simulink model "ex7p4"  (R2016b)
settings: Solver=VariableStepAuto  StartTime=0.0  StopTime=3  RelTol=1e-3
libraries: powerlib x9, simulink x1, powerlib_meascontrol x1
settings Model: Creator=user  LastModifiedBy=user

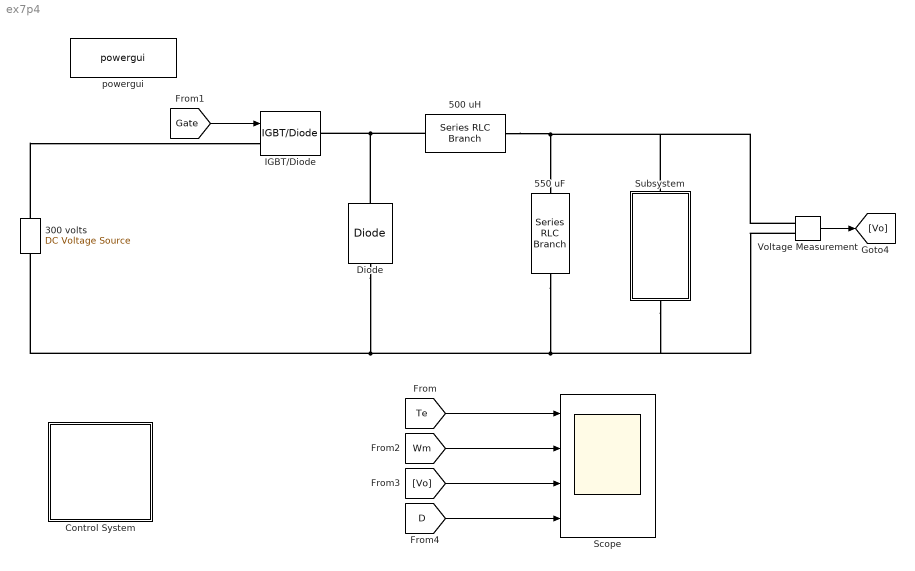
== system ex7p4 ==
  300 volts : powerlib/Electrical Sources/DC Voltage Source  Amplitude=300  Measurements=None
  500 uH : powerlib/Elements/Series RLC Branch  LConnTagsString=__new0  RConnTagsString=__new0  BranchType=L  Resistance=1  Inductance=500e-6  SetiL0=off  InitialCurrent=0  Capacitance=1e-6  Setx0=off  InitialVoltage=0  Measurements=None
  550 uF : powerlib/Elements/Series RLC Branch  LConnTagsString=__new0  RConnTagsString=__new0  BranchType=C  Resistance=1  Inductance=1e-3  SetiL0=off  InitialCurrent=0  Capacitance=550e-6  Setx0=on  InitialVoltage=150  Measurements=None
  "Control System " : Subsystem
  Diode : powerlib/Power Electronics/Diode  Ron=0.001  Lon=0  Vf=0.8  IC=0  UseSnubber=off  Rs=0  Cs=0  Measurements=off
  IGBT/Diode : powerlib/Power Electronics/IGBT//Diode  Ron=1e-3  Rs=1e5  Cs=inf  Measurements=off
  Scope : Scope  NumInputPorts=4
  Subsystem : Subsystem
  Voltage Measurement : powerlib/Measurements/Voltage Measurement  PhasorSimulation=off  OutputType=Complex  PSBequivalent=0
  powergui : powerlib/powergui  Priority=1  SimulationMode=Discrete  SolverType=Tustin/Backward Euler (TBE)  SampleTime=5e-6  frequency=60  SPID=off  DisableSnubberDevices=off  DisableRonSwitches=off  DisableVfSwitches=off  SwTol=0  DisplayEquations=off  Interpol=off  ExternalGateDelay=off  methode=off  Ts=10  FunctionMessages=off  echomessages=off  HookPort=off  EnableUseOfTLC=off  x0status=blocks  frequencyindice=0  Pbase=100e6  ErrMax=1e-4  Iterations=50  UnitsV=kV  UnitsW=MW  buscounter=0  RestoreLinks=warning  ResistiveCurrentMeasurement=off  Frange=[0:2:500]  Ylog=off  Xlog=on  ShowGrid=off  save=off  variable=ZData  structure=0  ZoomFFT=off  StartTime=0.0  cycles=1  DisplayStyle=1  fundamental=60  FreqAxis=off  MaxFrequency=1000  frequencyindicesteady=1  RmsSteady=1  display=off
  wires:
  Voltage Measurement/1 -> [Vo]
  [Te] -> Scope/1
  [Vo] -> Scope/3
  [D] -> Scope/4
  [Wm] -> Scope/2
  [Gate] -> IGBT/Diode/1
  connections:
  550 uF/RConn1 -- Subsystem/RConn1 -- Voltage Measurement/LConn2 -- Diode/LConn1 -- 300 volts/LConn1
  500 uH/LConn1 -- Subsystem/LConn1 -- Voltage Measurement/LConn1 -- 550 uF/LConn1
  300 volts/RConn1 -- IGBT/Diode/LConn1
  500 uH/RConn1 -- Diode/RConn1 -- IGBT/Diode/RConn1

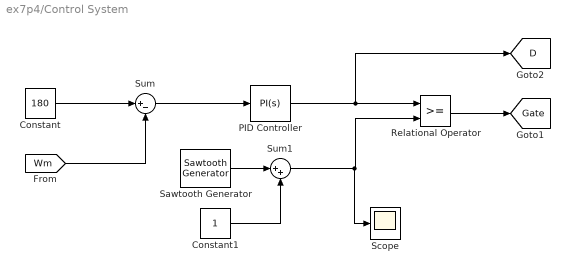
== system ex7p4/Control System  ==
  Constant : Constant  Value=180
  Constant1 : Constant
  PID Controller : simulink/Continuous/PID Controller  Controller=PI  TimeDomain=Continuous-time  SampleTime=-1  IntegratorMethod=Forward Euler  FilterMethod=Forward Euler  Form=Parallel  UseFilter=on  ControllerParametersSource=internal  P=0.1  I=2  D=0  N=100  InitialConditionSource=internal  InitialConditionForIntegrator=0  InitialConditionForFilter=0  ExternalReset=none  LimitOutput=off  UpperSaturationLimit=inf  LowerSaturationLimit=-inf  LinearizeAsGain=on  AntiWindupMode=none  Kb=1  TrackingMode=off  Kt=1  PParamMin=[]  PParamMax=[]  IParamMin=[]  IParamMax=[]  DParamMin=[]  DParamMax=[]  NParamMin=[]  NParamMax=[]  KbParamMin=[]  KbParamMax=[]  KtParamMin=[]  KtParamMax=[]  POutMin=[]  POutMax=[]  IOutMin=[]  IOutMax=[]  DOutMin=[]  DOutMax=[]  NOutMin=[]  NOutMax=[]  KbOutMin=[]  KbOutMax=[]  KtOutMin=[]  KtOutMax=[]  IntegratorOutMin=[]  IntegratorOutMax=[]  FilterOutMin=[]  FilterOutMax=[]  SumOutMin=[]  SumOutMax=[]  SumI1OutMin=[]  SumI1OutMax=[]  SumI2OutMin=[]  SumI2OutMax=[]  SumI3OutMin=[]  SumI3OutMax=[]  SumDOutMin=[]  SumDOutMax=[]  SaturationOutMin=[]  SaturationOutMax=[]  IntegratorContinuousStateAttributes=''  IntegratorStateMustResolveToSignalObject=off  IntegratorRTWStateStorageClass=Auto  FilterContinuousStateAttributes=''  FilterStateMustResolveToSignalObject=off  FilterRTWStateStorageClass=Auto  DifferentiatorICPrevScaledInput=0  DifferentiatorOutMin=[]  DifferentiatorOutMax=[]
  Relational Operator : RelationalOperator  OutDataTypeStr=boolean  RndMeth=Simplest
  Sawtooth Generator : powerlib_meascontrol/Pulse & Signal Generators/Sawtooth Generator  Freq=15000  Phase=0  Ts=0
  Scope : Scope
  Sum : Sum  Inputs=|+-
  Sum1 : Sum  Inputs=|++
  tag scope: D=global, Gate=global
  wires:
  Relational Operator/1 -> [Gate]
  Constant/1 -> Sum/1
  Sum1/1 -> Scope/1, Relational Operator/2
  Constant1/1 -> Sum1/2
  PID Controller/1 -> [D], Relational Operator/1
  Sawtooth Generator/1 -> Sum1/1
  [Wm] -> Sum/2
  Sum/1 -> PID Controller/1

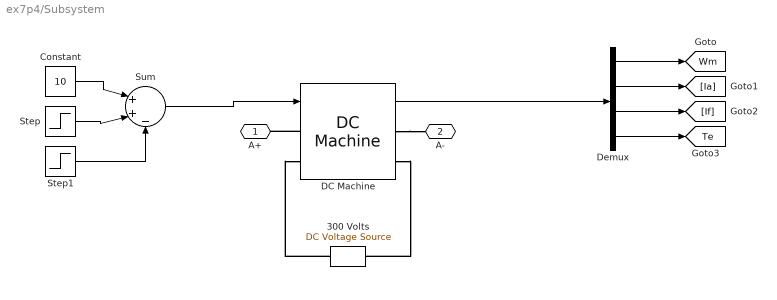
== system ex7p4/Subsystem ==
  300 Volts : powerlib/Electrical Sources/DC Voltage Source  Amplitude=300  Measurements=None
  Constant : Constant  Value=10
  DC Machine : powerlib/Machines/DC Machine  PresetModel=01: 5HP 240V 1750RPM Field:300V  MechanicalLoad=Torque TL  FieldType=Wound  ShowDetailedParameters=on  MeasurementBus=off  RLa=[2.581 0.028]  RLf=[281.3 156]  Laf=0.9483  MachineConstant=Torque constant (N.m/A)  Ke=1.8  Kt=1.8  J=0.02215  Bm=0.002953  Tf=0.5161  w0=1  Ifinit=1  TsPowergui=0  TsBlock=-1
  Demux : Demux
  Step : Step  After=10  SampleTime=0
  Step1 : Step  Time=2  After=10  SampleTime=0
  Sum : Sum  Inputs=|++-
  A+ : PMIOPort  Port=1  Side=Left
  A- : PMIOPort  Port=2  Side=Right
  tag scope: Te=global, Wm=global
  wires:
  Demux/2 -> [Ia]
  DC Machine/1 -> Demux/1
  Demux/1 -> [Wm]
  Constant/1 -> Sum/1
  Demux/3 -> [If]
  Demux/4 -> [Te]
  Sum/1 -> DC Machine/1
  Step/1 -> Sum/2
  Step1/1 -> Sum/3
  connections:
  DC Machine/RConn2 -- 300 Volts/LConn1
  DC Machine/LConn1 -- A+/RConn1
  DC Machine/RConn1 -- A-/RConn1
  300 Volts/RConn1 -- DC Machine/LConn2
